simulink model "AttitudeControl_tune"  (R2016b)
settings: Solver=ode4  StartTime=0.0  StopTime=10  FixedStep=0.001  RelTol=1e-3
InitFcn:
  | Init_control
values from neighbouring files (symbols this model uses):
  Kd_RP_AgngleRate = 0.001    [Init_control.m]
  Kd_YAW_AngleRate = 0.00    (= 0)    [Init_control.m]
  Ki_RP_AgngleRate = 0.02    [Init_control.m]
  Ki_YAW_AngleRate = 0.01    [Init_control.m]
  Kp_RP_AgngleRate = 0.10    (= 0.1)    [Init_control.m]
  Kp_RP_ANGLE = 6.5    [Init_control.m]
  Kp_YAW_AngleRate = 0.3    [Init_control.m]
  MAX_CONTROL_ANGLE_RATE_PITCH = 220    [Init_control.m]
  MAX_CONTROL_ANGLE_RATE_ROLL = 220    [Init_control.m]
  ModelInit_RPM = 557.1420    (= 557.142)    [Init_control.m]
  Saturation_I_RP_Max = 0.3    [Init_control.m]
  Saturation_I_RP_Min = -0.3    [Init_control.m]
  Saturation_I_Y_Max = 0.2    [Init_control.m]
  Saturation_I_Y_Min = -0.2    [Init_control.m]
undefined symbols (not defined in the file or in its folder): DiscIntNeverNeededParam, ModelParam_envGravityAcc, ModelParam_motorCr, ModelParam_motorJm, ModelParam_motorT, ModelParam_motorWb, ModelParam_rotorCm, ModelParam_rotorCt, ModelParam_uavCd, ModelParam_uavJ, ModelParam_uavMass, ModelParam_uavR
libraries: simulink x3, aerolibutil x2, aerolibtransform2 x1
settings Model: Creator=Mr Wang  LastModifiedBy=Mr Wang
settings OptimizationCC: MaxStackSize=64
settings DebuggingCC: ParameterTunabilityLossMsg=error
settings HardwareCC: ProdBitPerPointer=32  ProdBitPerSizeT=32  ProdBitPerPtrDiffT=32  ProdLargestAtomicInteger=Long  ProdLargestAtomicFloat=Double  ProdWordSize=32  ProdHWDeviceType=ARM Compatible->ARM Cortex
settings RTWCC: SystemTargetFile=ert.tlc  HardwareBoard=Pixhawk PX4  TLCOptions="-aInlineSetEventsForThisBaseRateFcn=TLC_FALSE -aSuppressMultiTaskScheduler=TLC_FALSE  -aRateBasedStepFcn=0"  TemplateMakefile=ert_default_tmf  Description=Embedded Coder  GenerateReport=on  Toolchain=Pixhawk Toolchain  IncludeHyperlinkInReport=on  LaunchReport=on  GenerateTraceInfo=on  GenerateTraceReport=on  GenerateTraceReportSl=on  GenerateTraceReportSf=on  GenerateTraceReportEml=on
settings CodeAppCC: ForceParamTrailComments=on  IgnoreCustomStorageClasses=off  OperatorAnnotations=on  SimulinkDataObjDesc=on  SFDataObjDesc=on  MATLABFcnDesc=on  InsertBlockDesc=on  MATLABSourceComments=on
settings ERTTargetCC: ERTCustomFileTemplate=PX4_codertarget_file_process.tlc

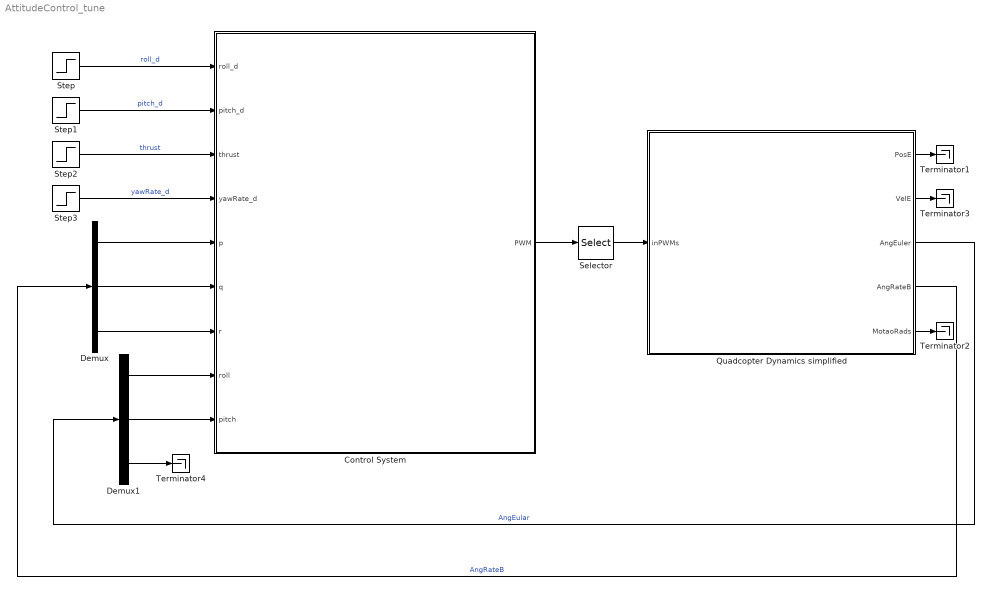
== system AttitudeControl_tune ==
  Control System : Subsystem
      mask Display: image('icon\pixhawk.png');
  Demux : Demux  Outputs=3
  Demux1 : Demux  Outputs=3
  "Quadcopter Dynamics simplified " : Subsystem
      mask Display: image('./icon/F450.png');
  Selector : Selector  InputPortWidth=8  IndexOptions=Index vector (dialog)  Indices=[1:4]  OutputSizes=1
  Step : Step  Time=0  After=0  SampleTime=0
  Step1 : Step  Time=0  After=0  SampleTime=0
  Step2 : Step  Time=0  After=0.6085  SampleTime=0
  Step3 : Step  Time=0  After=0  SampleTime=0
  Terminator{1..4} (4 alike) : Terminator
  wires:
  "Quadcopter Dynamics simplified "/3(AngEuler) -> Demux1/1  "AngEular"
  "Quadcopter Dynamics simplified "/4(AngRateB) -> Demux/1  "AngRateB"
  Demux/1 -> Control System/5(p)
  Demux/2 -> Control System/6(q)
  Demux/3 -> Control System/7(r)
  Demux1/1 -> Control System/8(roll)
  Demux1/3 -> Terminator4/1
  Demux1/2 -> Control System/9(pitch)
  "Quadcopter Dynamics simplified "/1(PosE) -> Terminator1/1
  Control System/1(PWM) -> Selector/1
  "Quadcopter Dynamics simplified "/2(VelE) -> Terminator3/1
  Selector/1 -> "Quadcopter Dynamics simplified "/1(inPWMs)
  Step1/1 -> Control System/2(pitch_d)  "pitch_d"
  Step/1 -> Control System/1(roll_d)  "roll_d"
  Step3/1 -> Control System/4(yawRate_d)  "yawRate_d"
  Step2/1 -> Control System/3(thrust)  "thrust"
  "Quadcopter Dynamics simplified "/5(MotaoRads) -> Terminator2/1

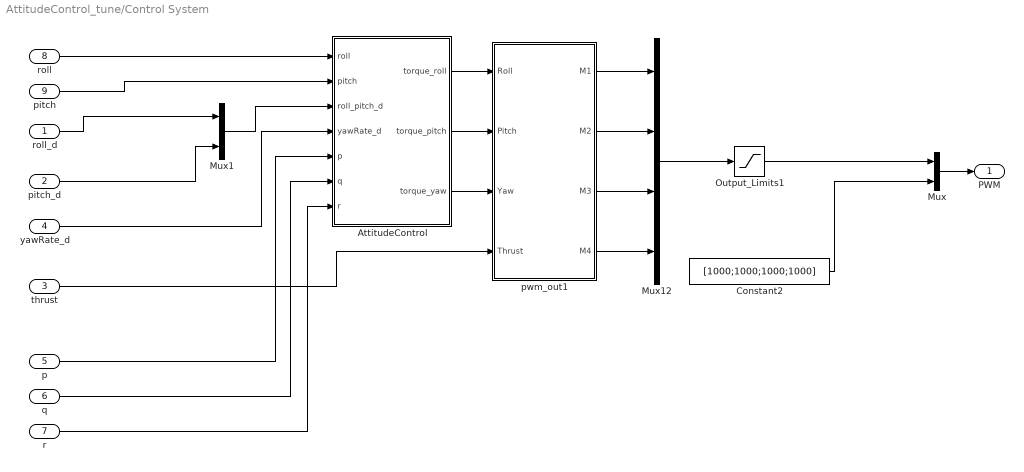
== system AttitudeControl_tune/Control System ==
  roll_d : Inport  PortDimensions=1
  pitch_d : Inport  Port=2  PortDimensions=1
  thrust : Inport  Port=3  PortDimensions=1
  yawRate_d : Inport  Port=4  PortDimensions=1
  p : Inport  Port=5  PortDimensions=1
  q : Inport  Port=6  PortDimensions=1
  r : Inport  Port=7  PortDimensions=1
  roll : Inport  Port=8  PortDimensions=1
  pitch : Inport  Port=9  PortDimensions=1
  AttitudeControl : Subsystem
  Constant2 : Constant  Value=[1000;1000;1000;1000]
  Mux : Mux  Inputs=2
  Mux1 : Mux  Inputs=2
  Mux12 : Mux
  Output_Limits1 : Saturate  UpperLimit=2000  LowerLimit=1000  LinearizeAsGain=off
  pwm_out1 : MATLAB Function  SystemSampleTime=0.004
  PWM : Outport
  wires:
  thrust/1 -> pwm_out1/4(Thrust)
  Mux12/1 -> Output_Limits1/1
  AttitudeControl/2(torque_pitch) -> pwm_out1/2(Pitch)
  AttitudeControl/1(torque_roll) -> pwm_out1/1(Roll)
  pwm_out1/1(M1) -> Mux12/1
  pwm_out1/3(M3) -> Mux12/3
  pwm_out1/2(M2) -> Mux12/2
  r/1 -> AttitudeControl/7(r)
  AttitudeControl/3(torque_yaw) -> pwm_out1/3(Yaw)
  Mux1/1 -> AttitudeControl/3(roll_pitch_d)
  q/1 -> AttitudeControl/6(q)
  yawRate_d/1 -> AttitudeControl/4(yawRate_d)
  p/1 -> AttitudeControl/5(p)
  pwm_out1/4(M4) -> Mux12/4
  pitch/1 -> AttitudeControl/2(pitch)
  roll/1 -> AttitudeControl/1(roll)
  Constant2/1 -> Mux/2
  Output_Limits1/1 -> Mux/1
  Mux/1 -> PWM/1
  roll_d/1 -> Mux1/1
  pitch_d/1 -> Mux1/2

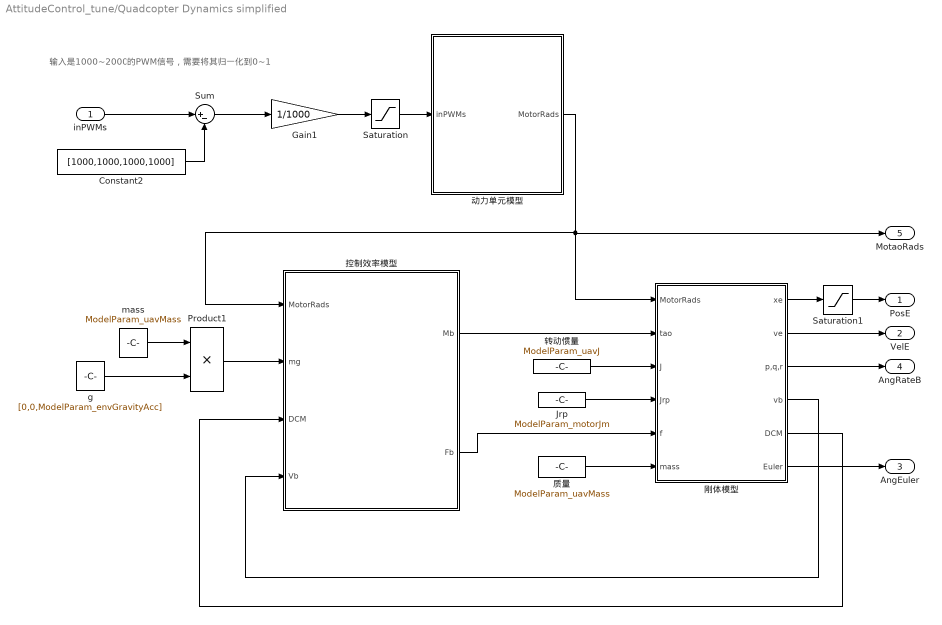
== system AttitudeControl_tune/Quadcopter Dynamics simplified  ==
  note: 输入是1000~2000的PWM信号，需要将其归一化到0~1
  inPWMs : Inport
  Constant2 : Constant  Value=[1000,1000,1000,1000]
  Gain1 : Gain  Gain=1/1000
  Jrp : Constant  Value=ModelParam_motorJm
  Product1 : Product
  Saturation : Saturate  UpperLimit=1  LowerLimit=0
  Saturation1 : Saturate  UpperLimit=[inf,inf,0]  LowerLimit=[-inf,-inf,-inf]
  Sum : Sum  Inputs=|+-
  g : Constant  Value=[0,0,ModelParam_envGravityAcc]
  mass : Constant  Value=ModelParam_uavMass
  刚体模型 : Subsystem
  动力单元模型 : Subsystem
  控制效率模型 : Subsystem
  质量 : Constant  Value=ModelParam_uavMass
  转动惯量 : Constant  Value=ModelParam_uavJ
  PosE : Outport
  VelE : Outport  Port=2
  AngEuler : Outport  Port=3
  AngRateB : Outport  Port=4
  MotaoRads : Outport  Port=5
  wires:
  g/1 -> Product1/2
  Constant2/1 -> Sum/2
  控制效率模型/2(Fb) -> 刚体模型/5(f)
  inPWMs/1 -> Sum/1
  控制效率模型/1(Mb) -> 刚体模型/2(tao)
  刚体模型/6(Euler) -> AngEuler/1
  Saturation1/1 -> PosE/1
  刚体模型/4("vb ") -> 控制效率模型/4(Vb)
  Product1/1 -> 控制效率模型/2(mg)
  Sum/1 -> Gain1/1
  刚体模型/2(ve) -> VelE/1
  Gain1/1 -> Saturation/1
  转动惯量/1 -> 刚体模型/3(J)
  动力单元模型/1(MotorRads) -> MotaoRads/1, 刚体模型/1(MotorRads), 控制效率模型/1(MotorRads)
  刚体模型/1("xe ") -> Saturation1/1
  刚体模型/5(DCM) -> 控制效率模型/3(DCM)
  mass/1 -> Product1/1
  质量/1 -> 刚体模型/6(mass)
  Jrp/1 -> 刚体模型/4(Jrp)
  刚体模型/3("p,q,r ") -> AngRateB/1
  Saturation/1 -> 动力单元模型/1(inPWMs)

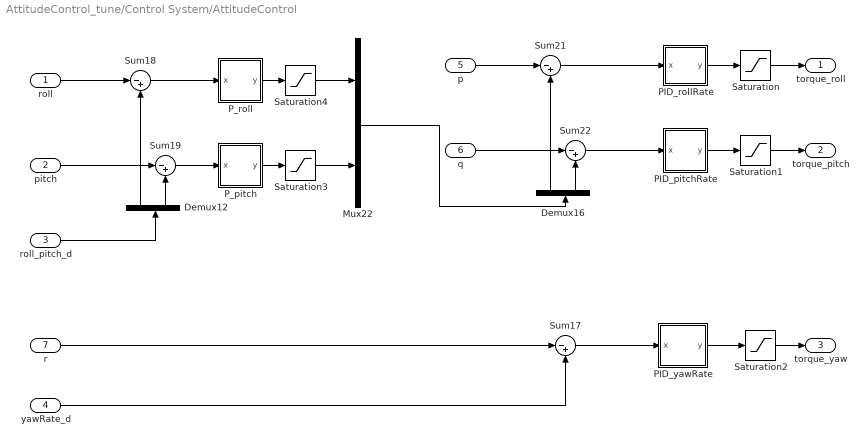
== system AttitudeControl_tune/Control System/AttitudeControl ==
  roll : Inport
  pitch : Inport  Port=2
  roll_pitch_d : Inport  Port=3
  yawRate_d : Inport  Port=4
  p : Inport  Port=5
  q : Inport  Port=6
  r : Inport  Port=7
  Demux12 : Demux  Outputs=2
  Demux16 : Demux  Outputs=2
  Mux22 : Mux  Inputs=2
  PID_pitchRate : Subsystem
  PID_rollRate : Subsystem
  PID_yawRate : Subsystem
  "P_pitch " : Subsystem
  "P_roll " : Subsystem
  Saturation : Saturate  UpperLimit=1  LowerLimit=-1
  Saturation1 : Saturate  UpperLimit=1  LowerLimit=-1
  Saturation2 : Saturate
  Saturation3 : Saturate  UpperLimit=MAX_CONTROL_ANGLE_RATE_PITCH  LowerLimit=-MAX_CONTROL_ANGLE_RATE_PITCH
  Saturation4 : Saturate  UpperLimit=MAX_CONTROL_ANGLE_RATE_ROLL  LowerLimit=-MAX_CONTROL_ANGLE_RATE_ROLL
  Sum{17..19,21..22} (5 alike) : Sum  Inputs=|-+
  torque_roll : Outport
  torque_pitch : Outport  Port=2
  torque_yaw : Outport  Port=3
  wires:
  r/1 -> Sum17/1
  Sum19/1 -> "P_pitch "/1(x)
  "P_pitch "/1(y) -> Saturation3/1
  "P_roll "/1(y) -> Saturation4/1
  roll/1 -> Sum18/1
  pitch/1 -> Sum19/1
  Sum18/1 -> "P_roll "/1(x)
  Sum22/1 -> PID_pitchRate/1(x)
  Sum17/1 -> PID_yawRate/1(x)
  p/1 -> Sum21/1
  q/1 -> Sum22/1
  Sum21/1 -> PID_rollRate/1(x)
  PID_pitchRate/1(y) -> Saturation1/1
  PID_rollRate/1(y) -> Saturation/1
  PID_yawRate/1(y) -> Saturation2/1
  roll_pitch_d/1 -> Demux12/1
  Saturation1/1 -> torque_pitch/1
  yawRate_d/1 -> Sum17/2
  Mux22/1 -> Demux16/1
  Saturation4/1 -> Mux22/1
  Saturation3/1 -> Mux22/2
  Saturation/1 -> torque_roll/1
  Saturation2/1 -> torque_yaw/1
  Demux16/1 -> Sum21/2
  Demux12/2 -> Sum19/2
  Demux12/1 -> Sum18/2
  Demux16/2 -> Sum22/2

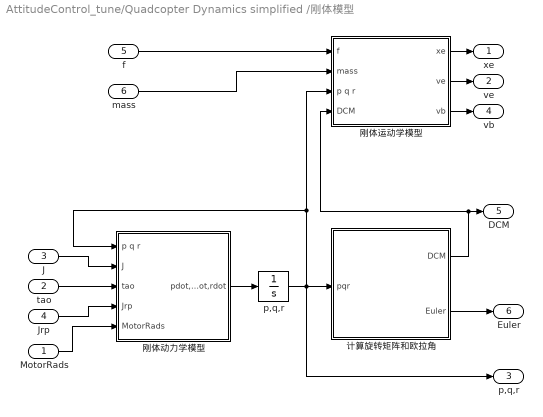
== system AttitudeControl_tune/Quadcopter Dynamics simplified /刚体模型 ==
  MotorRads : Inport
  tao : Inport  Port=2
  J : Inport  Port=3
  Jrp : Inport  Port=4
  f : Inport  Port=5
  mass : Inport  Port=6
  p,q,r : Integrator
  刚体动力学模型 : Subsystem
  刚体运动学模型 : Subsystem
  计算旋转矩阵和欧拉角 : Subsystem
  "xe " : Outport
  ve : Outport  Port=2
  "p,q,r " : Outport  Port=3
  "vb " : Outport  Port=4
  DCM : Outport  Port=5
  Euler : Outport  Port=6
  wires:
  J/1 -> 刚体动力学模型/2(J)
  tao/1 -> 刚体动力学模型/3(tao)
  Jrp/1 -> 刚体动力学模型/4(Jrp)
  MotorRads/1 -> 刚体动力学模型/5(MotorRads)
  刚体动力学模型/1(pdot,qdot,rdot) -> p,q,r/1
  计算旋转矩阵和欧拉角/1(DCM) -> DCM/1, 刚体运动学模型/4(DCM)
  计算旋转矩阵和欧拉角/2(Euler) -> Euler/1
  f/1 -> 刚体运动学模型/1(f)
  mass/1 -> 刚体运动学模型/2(mass)
  刚体运动学模型/1("xe ") -> "xe "/1
  刚体运动学模型/2(ve) -> ve/1
  p,q,r/1 -> 刚体运动学模型/3(p q r), 刚体动力学模型/1(p q r), "p,q,r "/1, 计算旋转矩阵和欧拉角/1(pqr)
  刚体运动学模型/3("vb ") -> "vb "/1

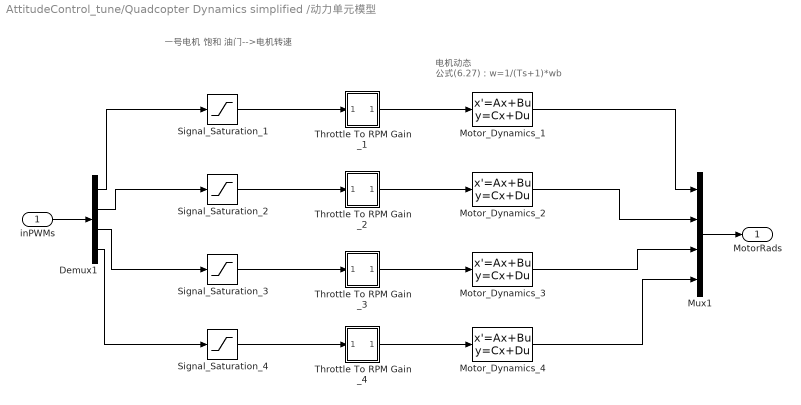
== system AttitudeControl_tune/Quadcopter Dynamics simplified /动力单元模型 ==
  note: 一号电机
      |
      |              饱和                             油门-->电机转速
  note: 电机动态
      | 公式(6.27)：w=1/(Ts+1)*wb
  inPWMs : Inport
  Demux1 : Demux
  Motor_Dynamics_{1..4} (4 alike) : StateSpace  A=-1/ModelParam_motorT  C=1/ModelParam_motorT  D=0  X0=ModelInit_RPM*ModelParam_motorT
  Mux1 : Mux
  Signal_Saturation_{1..4} (4 alike) : Saturate  UpperLimit=1  LowerLimit=0
  Throttle To RPM Gain _1 : Subsystem
  Throttle To RPM Gain _2 : Subsystem
  Throttle To RPM Gain _3 : Subsystem
  Throttle To RPM Gain _4 : Subsystem
  MotorRads : Outport
  wires:
  Demux1/1 -> Signal_Saturation_1/1
  Demux1/2 -> Signal_Saturation_2/1
  Demux1/3 -> Signal_Saturation_3/1
  Demux1/4 -> Signal_Saturation_4/1
  inPWMs/1 -> Demux1/1
  Throttle To RPM Gain _1/1(Out5) -> Motor_Dynamics_1/1
  Throttle To RPM Gain _2/1(Out5) -> Motor_Dynamics_2/1
  Throttle To RPM Gain _3/1(Out5) -> Motor_Dynamics_3/1
  Mux1/1 -> MotorRads/1
  Signal_Saturation_1/1 -> Throttle To RPM Gain _1/1(In5)
  Motor_Dynamics_1/1 -> Mux1/1
  Motor_Dynamics_2/1 -> Mux1/2
  Motor_Dynamics_3/1 -> Mux1/3
  Motor_Dynamics_4/1 -> Mux1/4
  Signal_Saturation_2/1 -> Throttle To RPM Gain _2/1(In5)
  Signal_Saturation_3/1 -> Throttle To RPM Gain _3/1(In5)
  Signal_Saturation_4/1 -> Throttle To RPM Gain _4/1(In5)
  Throttle To RPM Gain _4/1(Out5) -> Motor_Dynamics_4/1

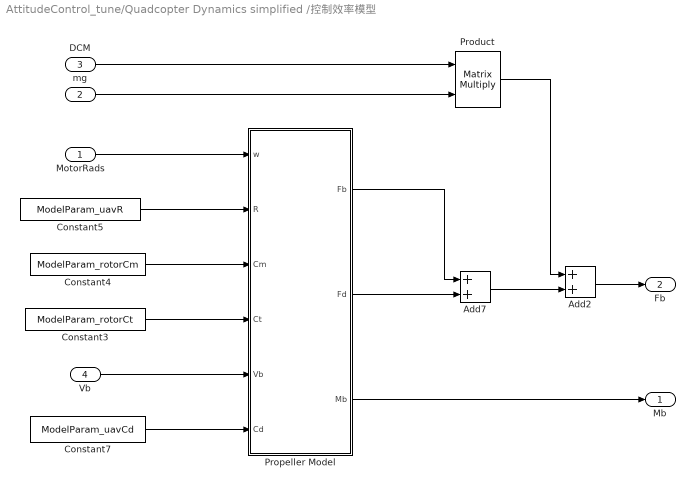
== system AttitudeControl_tune/Quadcopter Dynamics simplified /控制效率模型 ==
  MotorRads : Inport
  mg : Inport  Port=2
  DCM : Inport  Port=3
  Vb : Inport  Port=4
  Add2 : Sum
  Add7 : Sum
  Constant3 : Constant  Value=ModelParam_rotorCt
  Constant4 : Constant  Value=ModelParam_rotorCm
  Constant5 : Constant  Value=ModelParam_uavR
  Constant7 : Constant  Value=ModelParam_uavCd
  Product : Product  Multiplication=Matrix(*)
  Propeller Model : MATLAB Function  TreatAsAtomicUnit=on
  Mb : Outport
  Fb : Outport  Port=2
  wires:
  MotorRads/1 -> Propeller Model/1(w)
  Constant4/1 -> Propeller Model/3(Cm)
  Constant5/1 -> Propeller Model/2(R)
  Vb/1 -> Propeller Model/5(Vb)
  Constant7/1 -> Propeller Model/6(Cd)
  DCM/1 -> Product/1
  mg/1 -> Product/2
  Product/1 -> Add2/1
  Propeller Model/1(Fb) -> Add7/1
  Add7/1 -> Add2/2
  Propeller Model/2(Fd) -> Add7/2
  Constant3/1 -> Propeller Model/4(Ct)
  Add2/1 -> Fb/1
  Propeller Model/3(Mb) -> Mb/1

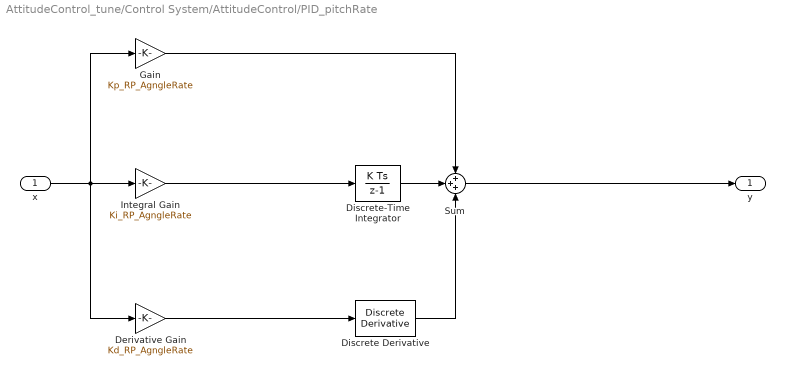
== system AttitudeControl_tune/Control System/AttitudeControl/PID_pitchRate ==
  x : Inport
  Derivative Gain : Gain  DisableCoverage=on  Gain=Kd_RP_AgngleRate  ParamMin=-100  ParamMax=100  OutMin=-100  OutMax=100
  Discrete Derivative : simulink/Discrete/Discrete Derivative  gainval=1.0  ICPrevScaledInput=0.0  OutMin=[]  OutMax=[]  OutDataType=fixdt(1, 16)  OutScaling=2^-10  DoSatur=off
  Discrete-Time Integrator : DiscreteIntegrator  InitialConditionSetting=State (most efficient)  SampleTime=-1  LimitOutput=on  UpperSaturationLimit=Saturation_I_RP_Max  LowerSaturationLimit=Saturation_I_RP_Min  ICPrevOutput=DiscIntNeverNeededParam  ICPrevScaledInput=DiscIntNeverNeededParam
  Gain : Gain  Gain=Kp_RP_AgngleRate
  Integral Gain : Gain  DisableCoverage=on  Gain=Ki_RP_AgngleRate
  Sum : Sum  Inputs=+++
  y : Outport  InitialOutput=0
  wires:
  Discrete-Time Integrator/1 -> Sum/2
  Discrete Derivative/1 -> Sum/3
  Sum/1 -> y/1
  Gain/1 -> Sum/1
  Derivative Gain/1 -> Discrete Derivative/1
  Integral Gain/1 -> Discrete-Time Integrator/1
  x/1 -> Derivative Gain/1, Integral Gain/1, Gain/1

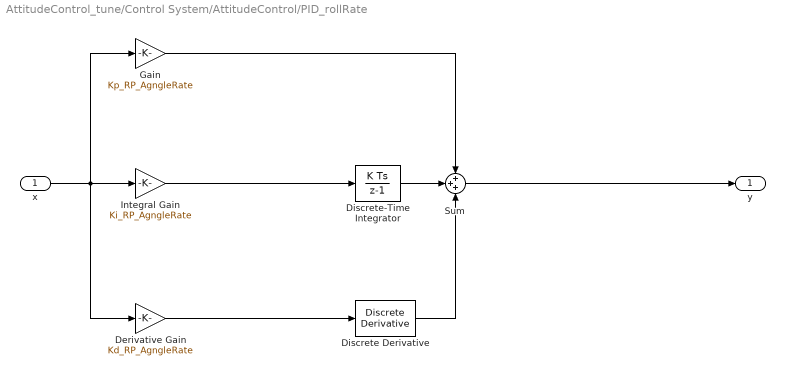
== system AttitudeControl_tune/Control System/AttitudeControl/PID_rollRate ==
  x : Inport
  Derivative Gain : Gain  DisableCoverage=on  Gain=Kd_RP_AgngleRate  ParamMin=-100  ParamMax=100  OutMin=-100  OutMax=100
  Discrete Derivative : simulink/Discrete/Discrete Derivative  gainval=1.0  ICPrevScaledInput=0.0  OutMin=[]  OutMax=[]  OutDataType=fixdt(1, 16)  OutScaling=2^-10  DoSatur=off
  Discrete-Time Integrator : DiscreteIntegrator  InitialConditionSetting=State (most efficient)  SampleTime=-1  LimitOutput=on  UpperSaturationLimit=Saturation_I_RP_Max  LowerSaturationLimit=Saturation_I_RP_Min  ICPrevOutput=DiscIntNeverNeededParam  ICPrevScaledInput=DiscIntNeverNeededParam
  Gain : Gain  Gain=Kp_RP_AgngleRate
  Integral Gain : Gain  DisableCoverage=on  Gain=Ki_RP_AgngleRate
  Sum : Sum  Inputs=+++
  y : Outport  InitialOutput=0
  wires:
  x/1 -> Gain/1, Integral Gain/1, Derivative Gain/1
  Integral Gain/1 -> Discrete-Time Integrator/1
  Derivative Gain/1 -> Discrete Derivative/1
  Gain/1 -> Sum/1
  Sum/1 -> y/1
  Discrete Derivative/1 -> Sum/3
  Discrete-Time Integrator/1 -> Sum/2

== system AttitudeControl_tune/Control System/AttitudeControl/PID_yawRate ==
  x : Inport
  Derivative Gain : Gain  DisableCoverage=on  Gain=Kd_YAW_AngleRate  ParamMin=-100  ParamMax=100  OutMin=-100  OutMax=100
  Discrete Derivative : simulink/Discrete/Discrete Derivative  gainval=1.0  ICPrevScaledInput=0.0  OutMin=[]  OutMax=[]  OutDataType=fixdt(1, 16)  OutScaling=2^-10  DoSatur=off
  Discrete-Time Integrator : DiscreteIntegrator  InitialConditionSetting=State (most efficient)  SampleTime=-1  LimitOutput=on  UpperSaturationLimit=Saturation_I_Y_Max  LowerSaturationLimit=Saturation_I_Y_Min  ICPrevOutput=DiscIntNeverNeededParam  ICPrevScaledInput=DiscIntNeverNeededParam
  Gain : Gain  Gain=Kp_YAW_AngleRate
  Integral Gain : Gain  DisableCoverage=on  Gain=Ki_YAW_AngleRate
  Sum : Sum  Inputs=+++
  y : Outport  InitialOutput=0
  wires:
  x/1 -> Gain/1, Integral Gain/1, Derivative Gain/1
  Integral Gain/1 -> Discrete-Time Integrator/1
  Derivative Gain/1 -> Discrete Derivative/1
  Gain/1 -> Sum/1
  Sum/1 -> y/1
  Discrete Derivative/1 -> Sum/3
  Discrete-Time Integrator/1 -> Sum/2

== system AttitudeControl_tune/Control System/AttitudeControl/P_pitch  ==
  x : Inport
  Gain : Gain  Gain=Kp_RP_ANGLE
  y : Outport  InitialOutput=0
  wires:
  x/1 -> Gain/1
  Gain/1 -> y/1

== system AttitudeControl_tune/Control System/AttitudeControl/P_roll  ==
  x : Inport
  Gain : Gain  Gain=Kp_RP_ANGLE
  y : Outport  InitialOutput=0
  wires:
  Gain/1 -> y/1
  x/1 -> Gain/1

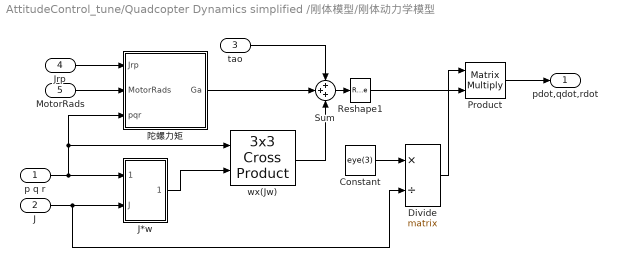
== system AttitudeControl_tune/Quadcopter Dynamics simplified /刚体模型/刚体动力学模型 ==
  p q r : Inport
  J : Inport  Port=2
  tao : Inport  Port=3
  Jrp : Inport  Port=4
  MotorRads : Inport  Port=5
  Constant : Constant  Value=eye(3)
  Divide : Product  Inputs=*/  Multiplication=Matrix(*)
  J*w : Subsystem
  Product : Product  Multiplication=Matrix(*)
  Reshape1 : Reshape  OutputDimensionality=Column vector (2-D)
  Sum : Sum  Inputs=3
  wx(Jw) : aerolibutil/3x3 Cross Product
  陀螺力矩 : MATLAB Function  TreatAsAtomicUnit=on
  pdot,qdot,rdot : Outport
  wires:
  wx(Jw)/1 -> Sum/3
  MotorRads/1 -> 陀螺力矩/2(MotorRads)
  Jrp/1 -> 陀螺力矩/1(Jrp)
  tao/1 -> Sum/1
  J*w/1("J*w ") -> wx(Jw)/2
  p q r/1 -> wx(Jw)/1, 陀螺力矩/3(pqr), J*w/1(p q r)
  J/1 -> J*w/2(J), Divide/2
  Sum/1 -> Reshape1/1
  Divide/1 -> Product/1
  陀螺力矩/1(Ga) -> Sum/2
  Constant/1 -> Divide/1
  Reshape1/1 -> Product/2
  Product/1 -> pdot,qdot,rdot/1

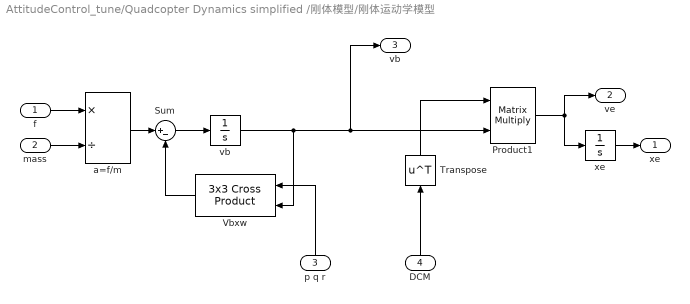
== system AttitudeControl_tune/Quadcopter Dynamics simplified /刚体模型/刚体运动学模型 ==
  f : Inport
  mass : Inport  Port=2
  p q r : Inport  Port=3
  DCM : Inport  Port=4
  Product1 : Product  Multiplication=Matrix(*)
  Sum : Sum  Inputs=|+-
  Transpose : Math  Operator=transpose  SaturateOnIntegerOverflow=on
  Vbxw : aerolibutil/3x3 Cross Product
  a=f/m : Product  Inputs=*/
  vb : Integrator
  xe : Integrator
  "xe " : Outport
  ve : Outport  Port=2
  "vb " : Outport  Port=3
  wires:
  DCM/1 -> Transpose/1
  p q r/1 -> Vbxw/1
  f/1 -> a=f/m/1
  Vbxw/1 -> Sum/2
  mass/1 -> a=f/m/2
  Transpose/1 -> Product1/1
  Product1/1 -> ve/1, xe/1
  xe/1 -> "xe "/1
  Sum/1 -> vb/1
  a=f/m/1 -> Sum/1
  vb/1 -> Vbxw/2, "vb "/1, Product1/2

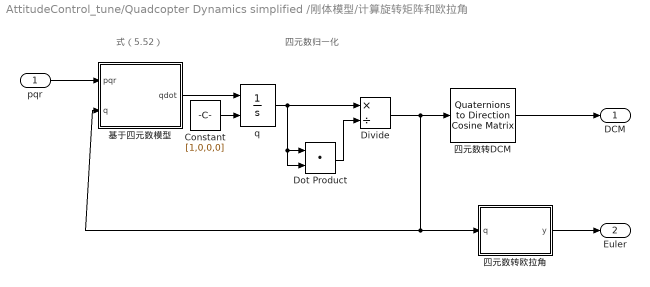
== system AttitudeControl_tune/Quadcopter Dynamics simplified /刚体模型/计算旋转矩阵和欧拉角 ==
  note: 四元数归一化
  note: 式（5.52）
  pqr : Inport
  Constant : Constant  Value=[1,0,0,0]
  Divide : Product  Inputs=*/
  Dot Product : DotProduct  InputSameDT=on  OutDataTypeStr=Inherit: Inherit via internal rule
  q : Integrator  InitialConditionSource=external
  四元数转DCM : aerolibtransform2/Quaternions to  Direction Cosine Matrix
  四元数转欧拉角 : MATLAB Function
  基于四元数模型 : MATLAB Function  TreatAsAtomicUnit=on
  DCM : Outport
  Euler : Outport  Port=2
  wires:
  Constant/1 -> q/2
  基于四元数模型/1(qdot) -> q/1
  q/1 -> Divide/1, Dot Product/2, Dot Product/1
  pqr/1 -> 基于四元数模型/1(pqr)
  四元数转DCM/1 -> DCM/1
  Dot Product/1 -> Divide/2
  Divide/1 -> 四元数转欧拉角/1(q), 基于四元数模型/2(q), 四元数转DCM/1
  四元数转欧拉角/1(y) -> Euler/1

== system AttitudeControl_tune/Quadcopter Dynamics simplified /动力单元模型/Throttle To RPM Gain _1 ==
  In5 : Inport
  Constant : Constant  Value=ModelParam_motorWb
  Gain : Gain  Gain=ModelParam_motorCr
  Sum1 : Sum  Inputs=++|
  Out5 : Outport
  wires:
  Sum1/1 -> Out5/1
  In5/1 -> Gain/1
  Gain/1 -> Sum1/2
  Constant/1 -> Sum1/1

== system AttitudeControl_tune/Quadcopter Dynamics simplified /动力单元模型/Throttle To RPM Gain _2 ==
  In5 : Inport
  Constant : Constant  Value=ModelParam_motorWb
  Gain : Gain  Gain=ModelParam_motorCr
  Sum1 : Sum  Inputs=++|
  Out5 : Outport
  wires:
  Constant/1 -> Sum1/1
  Gain/1 -> Sum1/2
  In5/1 -> Gain/1
  Sum1/1 -> Out5/1

== system AttitudeControl_tune/Quadcopter Dynamics simplified /动力单元模型/Throttle To RPM Gain _3 ==
  In5 : Inport
  Constant : Constant  Value=ModelParam_motorWb
  Gain : Gain  Gain=ModelParam_motorCr
  Sum1 : Sum  Inputs=++|
  Out5 : Outport
  wires:
  Sum1/1 -> Out5/1
  In5/1 -> Gain/1
  Gain/1 -> Sum1/2
  Constant/1 -> Sum1/1

== system AttitudeControl_tune/Quadcopter Dynamics simplified /动力单元模型/Throttle To RPM Gain _4 ==
  In5 : Inport
  Constant : Constant  Value=ModelParam_motorWb
  Gain : Gain  Gain=ModelParam_motorCr
  Sum1 : Sum  Inputs=++|
  Out5 : Outport
  wires:
  Constant/1 -> Sum1/1
  Gain/1 -> Sum1/2
  In5/1 -> Gain/1
  Sum1/1 -> Out5/1

== system AttitudeControl_tune/Quadcopter Dynamics simplified /刚体模型/刚体动力学模型/J*w ==
  p q r : Inport
  J : Inport  Port=2
  J*w : Product  Multiplication=Matrix(*)
  "J*w " : Outport
  wires:
  p q r/1 -> J*w/2
  J/1 -> J*w/1
  J*w/1 -> "J*w "/1

== matlab function AttitudeControl_tune/Quadcopter Dynamics simplified /刚体模型/刚体动力学模型/陀螺力矩 ==
  data: Jrp input; MotorRads input; pqr input; Ga output
function Ga = fcn(Jrp,MotorRads,pqr)
Ga=zeros(3,1);
Ga(1)=Jrp*pqr(2)*(-MotorRads(1)-MotorRads(2)+MotorRads(3)+MotorRads(4));
Ga(2)=Jrp*pqr(1)*( MotorRads(1)+MotorRads(2)-MotorRads(3)-MotorRads(4));

== matlab function AttitudeControl_tune/Quadcopter Dynamics simplified /刚体模型/计算旋转矩阵和欧拉角/基于四元数模型 ==
  data: pqr input; qdot output; q input
function qdot = fcn(pqr,q)

qdot=0.5*[0,-pqr(1),-pqr(2),-pqr(3);pqr(1),0,pqr(3),-pqr(2);pqr(2),-pqr(3),0,pqr(1);pqr(3),pqr(2),-pqr(1),0]*q;

== matlab function AttitudeControl_tune/Quadcopter Dynamics simplified /刚体模型/计算旋转矩阵和欧拉角/四元数转欧拉角 ==
  data: q input; y output
function y = fcn(q)

phi = atan2(2*(q(1)*q(2)+q(3)*q(4)),(1-2*(q(2)*q(2)+q(3)*q(3))));
theta = asin(2*(q(1)*q(3)-q(2)*q(4)));
psi = atan2(2*(q(1)*q(4)+q(2)*q(3)),(1-2*(q(3)*q(3))+q(4)*q(4)));
y = [phi theta psi];

== matlab function AttitudeControl_tune/Quadcopter Dynamics simplified /控制效率模型/Propeller Model ==
  data: w input; R input; Fb output; Fd output; Mb output; Cm input; Ct input; Vb input; Cd input
function [Fb,Fd,Mb] = fcn(w,R,Cm,Ct,Vb,Cd)
 %%叉字型
 %3  1
 %2  4
 M_rctcm = [-sin(pi/4)*R*Ct,sin(pi/4)*R*Ct,sin(pi/4)*R*Ct,-sin(pi/4)*R*Ct;
            sin(pi/4)*R*Ct,-sin(pi/4)*R*Ct,sin(pi/4)*R*Ct,-sin(pi/4)*R*Ct;
            Cm,Cm,-Cm,-Cm];
 Mb = M_rctcm*(w.^2);%式(6.24),力矩
 
 Fb = [0; 0; -sum(Ct*(w.^2))]; %(6.23),螺旋桨拉力
 Fd = -Cd*Vb.*abs(Vb)*0.5;%空气阻力
end

== matlab function AttitudeControl_tune/Control System/pwm_out1 ==
  data: Roll input; M1 output; Pitch input; Yaw input; Thrust input; M2 output; M3 output; M4 output
function [M1, M2, M3, M4] = motor_mixer(Roll, Pitch, Yaw, Thrust)
%quadrotorX
%3     1
%  \ /
%  / \
%2     4

idle_PWM = 1000;
scale = 1000;

M1 = (Thrust - Roll + Pitch + Yaw) * scale + idle_PWM;
M2 = (Thrust + Roll - Pitch + Yaw) * scale + idle_PWM;
M3 = (Thrust + Roll + Pitch - Yaw) * scale + idle_PWM;
M4 = (Thrust - Roll - Pitch - Yaw) * scale + idle_PWM;
